simulink model "lock"  (R2022b)
settings: Solver=FixedStepDiscrete  StartTime=0.0  StopTime=10.0  FixedStep=0.02  RelTol=1e-3
settings Model: Creator=ZhuanZ（无密码）  LastModifiedBy=ZhuanZ（无密码）
settings DataIOCC: SaveFormat=StructureWithTime
settings OptimizationCC: DefaultParameterBehavior=Inlined  EnhancedBackFolding=on  PassReuseOutputArgsAs=Individual arguments  ZeroExternalMemoryAtStartup=off  ZeroInternalMemoryAtStartup=off  OptimizeBlockOrder=speed  DifferentSizesBufferReuse=on  OptimizationCustomize=off  EfficientTunableParamExpr=on
settings DebuggingCC: ParameterTunabilityLossMsg=error
settings SFSimCC: MATLABDynamicMemAlloc=off
settings RTWCC: Description=AUTOSAR  SystemTargetFile=autosar.tlc  GenCodeOnly=on  TemplateMakefile=ert_default_tmf
settings CodeAppCC: ForceParamTrailComments=on  IgnoreCustomStorageClasses=off  OperatorAnnotations=on  SimulinkDataObjDesc=on  SFDataObjDesc=on  InsertBlockDesc=on
settings STFCustomTargetCC: TargetLangStandard=C99 (ISO)  MultiwordLength=256  ParMdlRefBuildCompliant=on  CompOptLevelCompliant=on  IncludeMdlTerminateFcn=off  CombineOutputUpdateFcns=on  SuppressErrorStatus=on  ERTCustomFileBanners=on  SupportNonFinite=off  SupportComplex=off  SupportContinuousTime=off  SupportNonInlinedSFcns=off  RemoveResetFunc=on  MATLABClassNameForMDSCustomization=Simulink.SoftwareTarget.ERTCustomization  AutosarCompliant=on  UseToolchainInfoCompliant=on  LookupTableObjectStructAxisOrder=2,1,3,4,...  LUTObjectStructOrderEvenSpacing=Size,Table,Breakpoints  SystemTargetFile=autosar.tlc
settings ERTTargetCC: TargetLangStandard=C99 (ISO)  ConcurrentExecutionCompliant=off  IncludeMdlTerminateFcn=off  SuppressErrorStatus=on  SupportNonFinite=off  SupportComplex=off  ModelStepFunctionPrototypeControlCompliant=off  CPPClassGenCompliant=off  AutosarCompliant=on  LookupTableObjectStructAxisOrder=2,1,3,4,...  LUTObjectStructOrderEvenSpacing=Size,Table,Breakpoints  InlinedParameterPlacement=NonHierarchical  ERTCustomFileTemplate=example_file_process.tlc

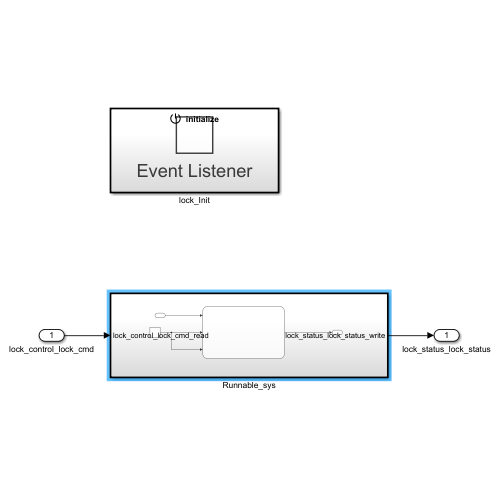
[thumbnail: Simulink's stored preview of the top-level diagram]
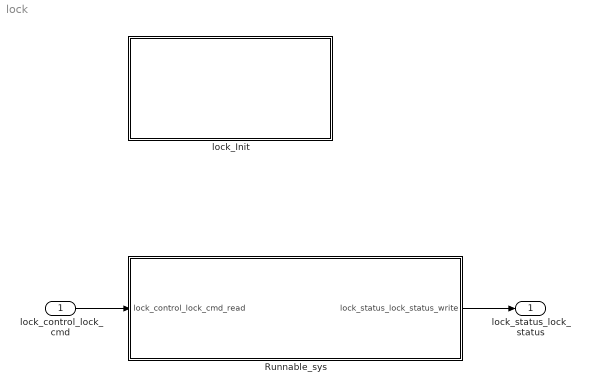
== system lock ==
  lock_control_lock_cmd : Inport  OutDataTypeStr=uint8  PortDimensions=1
  Runnable_sys : Subsystem  TreatAsAtomicUnit=on  SystemSampleTime=0.02
  lock_Init : Subsystem
  lock_status_lock_status : Outport  OutDataTypeStr=uint8  PortDimensions=1
  wires:
  lock_control_lock_cmd/1 -> Runnable_sys/1(lock_control_lock_cmd_read)
  Runnable_sys/1(lock_status_lock_status_write) -> lock_status_lock_status/1

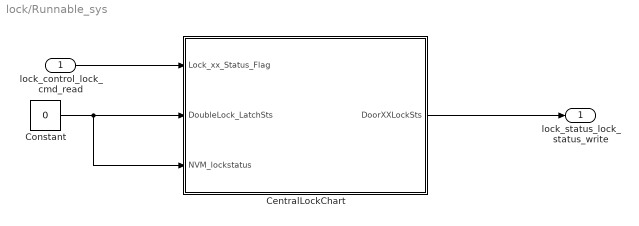
== system lock/Runnable_sys ==
  lock_control_lock_cmd_read : Inport
  CentralLockChart : Stateflow chart  TreatAsAtomicUnit=on
  Constant : Constant  Value=0  OutDataTypeStr=uint8
  lock_status_lock_status_write : Outport
  wires:
  lock_control_lock_cmd_read/1 -> CentralLockChart/1(Lock_xx_Status_Flag)
  CentralLockChart/1(DoorXXLockSts) -> lock_status_lock_status_write/1
  Constant/1 -> CentralLockChart/3(NVM_lockstatus), CentralLockChart/2(DoubleLock_LatchSts)

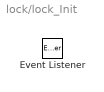
== system lock/lock_Init ==
  Event Listener : EventListener  EventName=reset

== stateflow chart lock/Runnable_sys/CentralLockChart ==
  state LockStsUkwn
    en:
    DoorXXLockSts = 0;%LockSts2_3.LockSts2_LockStsUkwn
  state Lock
    en:
    DoorXXLockSts =1;%LockSts2_3.LockSts2_Lockd
  state Unlock
    en:
    DoorXXLockSts = 2;%LockSts2_3.LockSts2_Unlckd
  state SafeLock
    en:
    DoorXXLockSts =3;%LockSts2_3.LockSts2_SafeLockd
  (default) -> LockStsUkwn
  LockStsUkwn -> (junction 17) [order 1] : [(Lock_xx_Status_Flag == 1)||...
      | (NVM_lockstatus == 1)]
  LockStsUkwn -> (junction 19) [order 2]
  (junction 17) -> Lock
  (junction 19) -> Unlock
  Unlock -> Lock : [Lock_xx_Status_Flag == 1]
  Lock -> Unlock [order 1] : [Lock_xx_Status_Flag ==2]
  Lock -> SafeLock [order 2] : [DoubleLock_LatchSts == 1]
  SafeLock -> Unlock : [(DoubleLock_LatchSts == 0 )&&(Lock_xx_Status_Flag ==2)]
  data: Lock_xx_Status_Flag input; DoorXXLockSts output uint8; DoubleLock_LatchSts input; NVM_lockstatus input
